simulink model "bangBangControl2018a"  (R2018a)
settings: Solver=VariableStepAuto  StartTime=0.0  StopTime=10.0  RelTol=1e-3
settings Model: Creator=mpi  LastModifiedBy=mpi

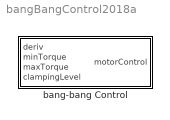
== system bangBangControl2018a ==
  bang-bang Control : MATLAB Function  TreatAsAtomicUnit=on

== matlab function bangBangControl2018a/bang-bang Control ==
  data: deriv input; motorControl output; minTorque input; maxTorque input; clampingLevel input
function motorControl   = fcn(deriv,minTorque, maxTorque, clampingLevel)
    persistent  drive lastDeriv signDeriv clamping;
    if(isempty(drive))
        drive = int16(15);
        lastDeriv = 0;
        signDeriv = 0;
        clamping = 0;
    end

    if(deriv==0)
        if(~clamping)
            if(lastDeriv > 0)
                drive = int16(maxTorque);
            else
                drive = int16(minTorque);
            end
            clamping = 1;
            signDeriv = lastDeriv;
        end
    end
    
    if(clamping)
        if(signDeriv > 0 && deriv < (-1 * clampingLevel))
            clamping  = 0;
        elseif(signDeriv < 0 && deriv > clampingLevel)
            clamping = 0;
        end
    end
    
    lastDeriv = deriv;
    motorControl = double(drive);
